simulink model "ur10_virtual_jointspace"  (R2025b)
settings: Solver=FixedStepDiscrete  StartTime=0.0  StopTime=10  FixedStep=0.02  RelTol=1e-3
undefined symbols (not defined in the file or in its folder): estimate_current_simple, virtual_ur10_alpha, virtual_ur10_current_bias, virtual_ur10_current_gain_ddq, virtual_ur10_current_gain_dq, virtual_ur10_current_gain_q, virtual_ur10_motor_gains
libraries: simulink x2
settings Model: Creator=18262  LastModifiedBy=18262

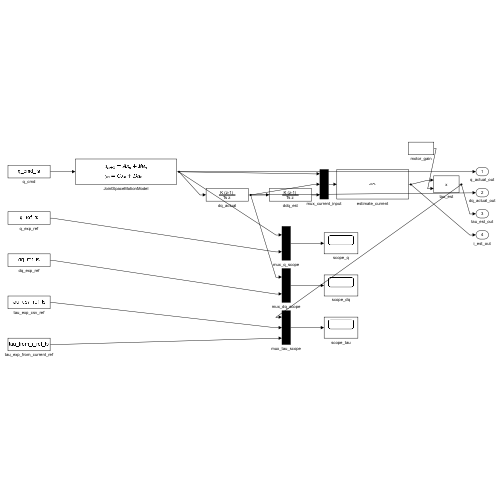
[thumbnail: Simulink's stored preview of the top-level diagram]
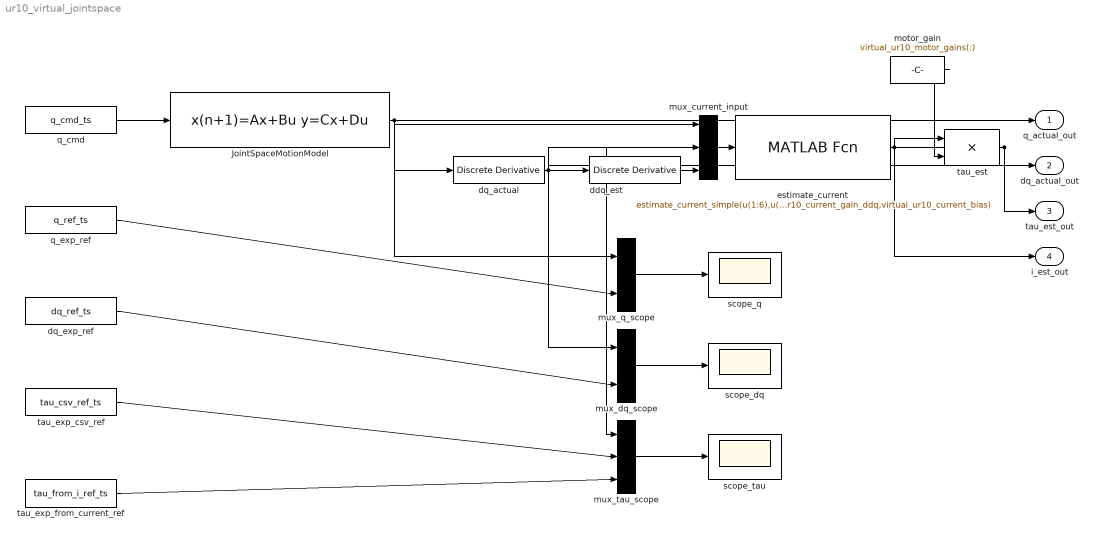
== system ur10_virtual_jointspace ==
  JointSpaceMotionModel : DiscreteStateSpace  A=(1-virtual_ur10_alpha)*eye(6)  B=virtual_ur10_alpha*eye(6)  C=eye(6)  D=zeros(6)  InitialCondition=zeros(6,1)  SampleTime=-1
  ddq_est : simulink/Discrete/Discrete Derivative  gainval=1/0.02  ICPrevScaledInput=0  OutMin=[]  OutMax=[]  OutDataType=fixdt(1, 16)  OutScaling=2^-10  DoSatur=off
  dq_actual : simulink/Discrete/Discrete Derivative  gainval=1/0.02  ICPrevScaledInput=0  OutMin=[]  OutMax=[]  OutDataType=fixdt(1, 16)  OutScaling=2^-10  DoSatur=off
  dq_exp_ref : FromWorkspace  VariableName=dq_ref_ts
  estimate_current : MATLABFcn  MATLABFcn=estimate_current_simple(u(1:6),u(7:12),u(13:18),virtual_ur10_current_gain_q,virtual_ur10_current_gain_dq,virtual_ur10_current_gain_ddq,virtual_ur10_current_bias)
  motor_gain : Constant  Value=virtual_ur10_motor_gains(:)
  mux_current_input : Mux  Inputs=3
  mux_dq_scope : Mux  Inputs=2
  mux_q_scope : Mux  Inputs=2
  mux_tau_scope : Mux  Inputs=3
  q_cmd : FromWorkspace  VariableName=q_cmd_ts
  q_exp_ref : FromWorkspace  VariableName=q_ref_ts
  scope_dq : Scope
  scope_q : Scope
  scope_tau : Scope
  tau_est : Product
  tau_exp_csv_ref : FromWorkspace  VariableName=tau_csv_ref_ts
  tau_exp_from_current_ref : FromWorkspace  VariableName=tau_from_i_ref_ts
  q_actual_out : Outport  PortDimensions=6
  dq_actual_out : Outport  Port=2  PortDimensions=6
  tau_est_out : Outport  Port=3  PortDimensions=6
  i_est_out : Outport  Port=4  PortDimensions=6
  wires:
  q_cmd/1 -> JointSpaceMotionModel/1
  JointSpaceMotionModel/1 -> dq_actual/1, mux_current_input/1, q_actual_out/1, mux_q_scope/1
  dq_actual/1 -> ddq_est/1, mux_current_input/2, dq_actual_out/1, mux_dq_scope/1
  ddq_est/1 -> mux_current_input/3
  mux_current_input/1 -> estimate_current/1
  estimate_current/1 -> tau_est/1, i_est_out/1
  motor_gain/1 -> tau_est/2
  tau_est/1 -> tau_est_out/1, mux_tau_scope/1
  q_exp_ref/1 -> mux_q_scope/2
  dq_exp_ref/1 -> mux_dq_scope/2
  tau_exp_csv_ref/1 -> mux_tau_scope/2
  tau_exp_from_current_ref/1 -> mux_tau_scope/3
  mux_q_scope/1 -> scope_q/1
  mux_dq_scope/1 -> scope_dq/1
  mux_tau_scope/1 -> scope_tau/1
